simulink model "eTRU_prototype_2"  (R2021b)
settings: Solver=daessc  StartTime=0.0  StopTime=5000  MaxStep=1  RelTol=1e-2  AbsTol=1e-2
PostLoadFcn:
  | eTRU_prototype_2_init
InitFcn:
  | eTRU_prototype_2_start_sim
StartFcn:
  | tic
StopFcn:
  | toc
  | PlotSimResults
values from neighbouring files (symbols this model uses):
  AirFlow = [0 0 0 0 0 0 0 0 0 0;      2205 1950 1701 1679 1297 658 0 0 0 0;      2989 2767 2610 2594 2410 2343 2274 1771 0 0;      3704 3545 3432 3422 3307 3266 3216 2958 2888 2215]    [EC_FanData.m]
  ambient_temp = 20    [eTRU_prototype_2_start_sim.m]
  asm = block.DialogPrm(1).Data    [msfcn_StaticASM.m]
  box_start_temp = 20    [eTRU_prototype_2_start_sim.m]
  cargo_start_temp = box_start_temp    (= 20)    [eTRU_prototype_2_start_sim.m]
  Power = [5 5 5 5 5 5 5 5 5 5;      185 203 227 226 229 230 231 237 239 247;      420 442 458 461 496 509 522 528 530 538;      764 811 844 846 880 892 905 969 987 989]    [EC_FanData.m]
  Pressure = LimitValue(Pressure + LimitValue(Error/dvdP, -0.1, 0.1), obj.PressureMin/100000, obj.PressureMax/100000)    [CoolPropPyWrapper.m]    (also in EC_FanData.m = [0,127,217,225,316,349,383,559,607,865])
  Speed = [0,1840,2450,3060]    [EC_FanData.m]
libraries: fl_lib x109, nesl_utility x82, simulink_extras x13, SimscapeFluids_lib x4
(part 1 of 3)
settings Model: Creator=kks  LastModifiedBy=kaspe
settings SolverCC: MaxConsecutiveMinStep=1000  AlgebraicLoopSolver=TrustRegion
settings DataIOCC: SaveState=on
settings DebuggingCC: ReadBeforeWriteMsg=DisableAll  WriteAfterWriteMsg=DisableAll  WriteAfterReadMsg=DisableAll  MultiTaskDSMMsg=none  SFMachineParentedDataDiag=warning
settings ModelReferenceCC: UpdateModelReferenceTargets=IfOutOfDate
settings SFSimCC: SFSimEcho=off
settings SimscapeCC: SimscapeLogLimitData=off

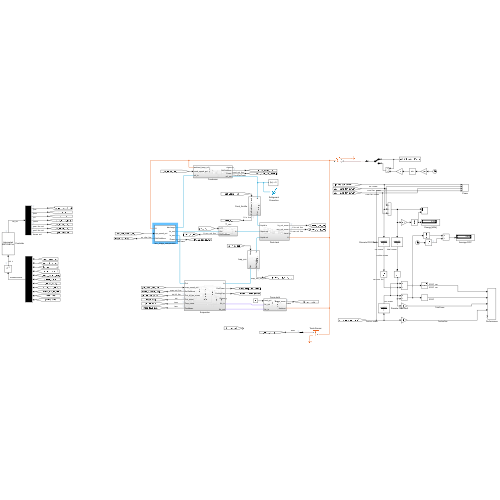
[thumbnail: Simulink's stored preview of the top-level diagram]
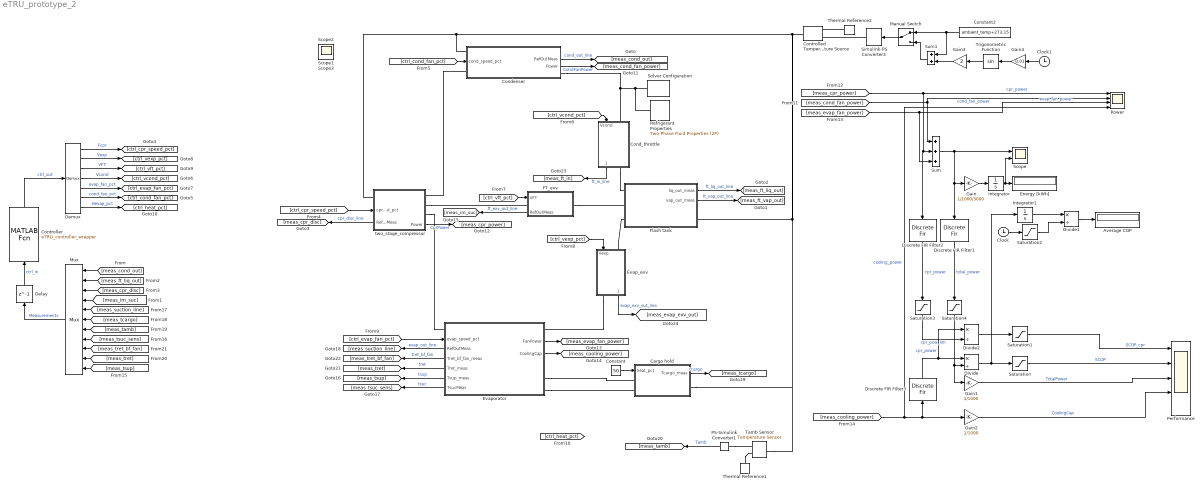
== system eTRU_prototype_2 ==
  Average COP : Display
  Cargo hold : Subsystem
  Clock : Clock
  Clock1 : Clock
  Cond_throttle : Subsystem
  Condenser : Subsystem
      settings: PortSchema="{\"entries\":[{\"content\":{\"sides\":[{\"content\":{\"connectorIds\":[\"LConn1\",\"In1\",\"LConn2\"]},\"type\":\"ConnectorPlacement.EquallySpacedRectSide\",\"uuid\":\"3d48dd4d-d64c-4c15-b87d-785ca519fd3e\"},{\"content\":{\"connectorIds\":[\"RConn1\",\"Out1\",\"Out2\",\"RConn2\"],\"side\":\"RIGHT\"},\"type\":\"ConnectorPlacement.EquallySpacedRectSide\",\"uuid\":\"adb43978-d4cf-4a53-b69c-b8e1726fc973\"},{\"content\":{\"connectorIds\":[],\"side\":\"TOP\"},\"type\":\"ConnectorPlacement.EquallySpacedRectSide\",\"uuid\":\"eda02cea-398b-4f5b-b755-168cdb387b03\"}]},\"type\":\"ConnectorPlacement.EquallySpacedConnector\",\"uuid\":\"bc915acd-4d9f-4179-86b8-14e03912b6e2\"}],\"packageUris\":[\"http://schema.mathworks.com/mf0/Connector/19700101\"],\"version\":\"1.0\"}"
  Constant : Constant  Value=50
  Constant2 : Constant  Value=ambient_temp+273.15
  Controlled Temperature Source : fl_lib/Thermal/Thermal Sources/Controlled Temperature Source
  Controller : MATLABFcn  StartFcn=eTRU_prototype_2_start_sim  MATLABFcn=eTRU_controller_wrapper
  Delay : Delay  DelayLength=1  InitialCondition=0  SampleTime=1
  Demux : Demux  Outputs=7
  Discrete FIR Filter1 : DiscreteFir  Coefficients=ones(1,300)/300
  Discrete FIR Filter2 : DiscreteFir  Coefficients=ones(1,300)/300
  Discrete FIR Filter3 : DiscreteFir  Coefficients=ones(1,300)/300
  Divide : Product  Inputs=*/
  Divide1 : Product  Inputs=*/
  Divide2 : Product  Inputs=*/
  Energy [kWh] : Display
  Evap_exv : Subsystem
      settings: PortSchema="{\"entries\":[{\"content\":{\"sides\":[{\"content\":{\"connectorIds\":[\"In1\",\"LConn1\"]},\"type\":\"ConnectorPlacement.EquallySpacedRectSide\",\"uuid\":\"a5f6ab4e-c003-4b63-bc8d-93a191bbc7b1\"},{\"content\":{\"connectorIds\":[\"RConn1\",\"Out1\"],\"side\":\"RIGHT\"},\"type\":\"ConnectorPlacement.EquallySpacedRectSide\",\"uuid\":\"60081e7c-9034-44ee-b85a-7fac1643604f\"},{\"content\":{\"connectorIds\":[],\"side\":\"TOP\"},\"type\":\"ConnectorPlacement.EquallySpacedRectSide\",\"uuid\":\"44f742ed-3697-4889-bc61-109290b38d73\"}]},\"type\":\"ConnectorPlacement.EquallySpacedConnector\",\"uuid\":\"b280b62a-8ac3-4a4b-85e3-fe929e92acc5\"}],\"packageUris\":[\"http://schema.mathworks.com/mf0/Connector/19700101\"],\"version\":\"1.0\"}"
  Evaporator : Subsystem
      settings: PortSchema="{\"entries\":[{\"content\":{\"sides\":[{\"content\":{\"connectorIds\":[\"LConn1\",\"In1\",\"Out3\",\"Out4\",\"Out5\",\"Out6\",\"Out7\"]},\"type\":\"ConnectorPlacement.EquallySpacedRectSide\",\"uuid\":\"033e4ee9-ae46-49ce-a29c-cb5691fe85b1\"},{\"content\":{\"connectorIds\":[\"RConn1\",\"Out1\",\"Out2\",\"RConn2\",\"RConn3\",\"RConn4\"],\"side\":\"RIGHT\"},\"type\":\"ConnectorPlacement.EquallySpacedRectSide\",\"uuid\":\"f5a957f7-d19d-4090-8dc6-9509ce363ce4\"},{\"content\":{\"connectorIds\":[],\"side\":\"TOP\"},\"type\":\"ConnectorPlacement.EquallySpacedRectSide\",\"uuid\":\"205ae6f2-ec5f-44bf-8412-6f03b41c638f\"},{\"content\":{\"connectorIds\":[],\"side\":\"BOTTOM\"},\"type\":\"ConnectorPlacement.EquallySpacedRectSide\",\"uuid\":\"b2e4c10a-8ecc-4b98-af22-93916696f813\"}]},\"type\":\"ConnectorPlacement.EquallySpacedConnector\",\"uuid\":\"b34f6f4b-92a6-4590-84b6-895e3d79e9bc\"}],\"packageUris\":[\"http://schema.mathworks.com/mf0/Connector/19700101\"],\"version\":\"1.0\"}"
  FT_exv : Subsystem
      settings: PortSchema="{\"entries\":[{\"content\":{\"sides\":[{\"content\":{\"connectorIds\":[\"LConn1\"]},\"type\":\"ConnectorPlacement.EquallySpacedRectSide\",\"uuid\":\"b279e9a8-1d21-4470-93a8-fbc83ce7b0b2\"},{\"content\":{\"connectorIds\":[\"In1\",\"RConn1\",\"Out1\"],\"side\":\"RIGHT\"},\"type\":\"ConnectorPlacement.EquallySpacedRectSide\",\"uuid\":\"0dfd93ae-010b-42e4-9e53-34ca9fdad0fd\"},{\"content\":{\"connectorIds\":[],\"side\":\"TOP\"},\"type\":\"ConnectorPlacement.EquallySpacedRectSide\",\"uuid\":\"f2d96627-f93b-40b5-bdbb-54ea25241c46\"}]},\"type\":\"ConnectorPlacement.EquallySpacedConnector\",\"uuid\":\"5e92ae64-a64b-485f-9000-97fefa6ea4c6\"}],\"packageUris\":[\"http://schema.mathworks.com/mf0/Connector/19700101\"],\"version\":\"1.0\"}"
  Flash tank : Subsystem
  Gain : Gain  Gain=1/1000/3600
  Gain1 : Gain  Gain=1/1000
  Gain2 : Gain  Gain=1/1000
  Gain3 : Gain  Gain=2
  Gain4 : Gain  Gain=0.01
  Integrator : Integrator
  Integrator1 : Integrator
  Manual Switch : ManualSwitch
  Mux : Mux  Inputs=11
  PS-Simulink Converter1 : nesl_utility/PS-Simulink Converter  PhysicalDomain=network_engine_domain  SubClassName=ps_output  LeftPortType=input  RightPortType=output  PseudoPeriodic=off  Frequencies=[]  Unit=inherit  AffineConversion=off
      settings: SourceProductBaseCode=PW,SS
  Performance : Scope  NumInputPorts=5
  Power : Scope  NumInputPorts=4
  Refrigerant Properties : fl_lib/Two-Phase Fluid/Utilities/Two-Phase Fluid Properties (2P)  u_min=RefrigerantPropertyTables.u_min kJ/kg  u_max=RefrigerantPropertyTables.u_max kJ/kg  p_TLU=RefrigerantPropertyTables.p MPa  p_crit=RefrigerantPropertyTables.p_crit MPa  critical_region=foundation.enum.critical_region.clip  p_crit_fraction=0.12  p_atm=0.101325 MPa  q_rev=0.01 Pa  unorm_liq=RefrigerantPropertyTables.liquid.unorm  v_liq=RefrigerantPropertyTables.liquid.v m^3/kg  s_liq=RefrigerantPropertyTables.liquid.s kJ/(K*kg)  T_liq=RefrigerantPropertyTables.liquid.T K  nu_liq=RefrigerantPropertyTables.liquid.nu mm^2/s  k_liq=RefrigerantPropertyTables.liquid.k W/(m*K)  Pr_liq=RefrigerantPropertyTables.liquid.Pr  u_sat_liq=RefrigerantPropertyTables.liquid.u_sat kJ/kg  unorm_vap=RefrigerantPropertyTables.vapor.unorm  v_vap=RefrigerantPropertyTables.vapor.v m^3/kg  s_vap=RefrigerantPropertyTables.vapor.s kJ/(K*kg)  T_vap=RefrigerantPropertyTables.vapor.T K  nu_vap=RefrigerantPropertyTables.vapor.nu mm^2/s  k_vap=RefrigerantPropertyTables.vapor.k W/(m*K)  Pr_vap=RefrigerantPropertyTables.vapor.Pr  u_sat_vap=RefrigerantPropertyTables.vapor.u_sat kJ/kg
      settings: SourceProductBaseCode=SS  InternalSimscapePortConfiguration="{\"Bottom\":[],\"Left\":[],\"Right\":[{\"id\":\"A\",\"label\":\"\",\"type\":\"foundation.two_phase_fluid.two_phase_fluid\"}],\"Top\":[]}"
  Saturation : Saturate  UpperLimit=10  LowerLimit=0
  Saturation1 : Saturate  UpperLimit=10  LowerLimit=0
  Saturation2 : Saturate  UpperLimit=20000000  LowerLimit=0.0001
  Saturation3 : Saturate  UpperLimit=20000  LowerLimit=0.0001
  Saturation4 : Saturate  UpperLimit=20000  LowerLimit=0.0001
  Scope : Scope  NumInputPorts=2
  Simulink-PS Converter3 : nesl_utility/Simulink-PS Converter  PhysicalDomain=network_engine_domain  SubClassName=ps_input  LeftPortType=input  RightPortType=output  PseudoPeriodic=off  Frequencies=[]  NoiseDistribution=none  NoiseParameters=[]  Unit=K  AffineConversion=off  FilteringAndDerivatives=zero  SimscapeFilterOrder=1  InputFilterTimeConstant=0.001  UdotUserProvided=1
      settings: SourceProductBaseCode=PW,SS
  Solver Configuration : nesl_utility/Solver Configuration  PhysicalDomain=network_engine_domain  SubClassName=solver  LeftPortType=input  RightPortType=generic  Tones=[]  Harmonics=[]  SimulateNoise=off  Profile=off  UseLocalSampling=off  EnableSwitchedLinearOptims=on  FrequencyDomain=off  UseCCode=off  RelTol=0.001  AbsTol=1e-06  MinStep=1e-09  ToWorkspace=off  RevertToSquareIcSolve=off  NumHomotopyIterations=100  PhasorMode=off  PhasorModeNumHarmonics=1  DoDC=off  ResidualTolerance=1e-3  UseLocalSolver=off  LocalSolverChoice=NE_BACKWARD_EULER_ADVANCER  LocalSolverSampleTime=.01  DoFixedCost=off  MaxNonlinIter=3  MaxModeIter=2  ComputeImpulses=off  ImpulseIterations=2  LinearAlgebra=auto  EquationFormulation=NE_TIME_EF  DelaysMemoryBudget=1024  AutomaticFiltering=on  FilteringTimeConstant=0.001  PartitionStorageMethod=AS_NEEDED  PartitionMemoryBudget=1024  PartitionMethod=FAST
      settings: SourceProductBaseCode=PW,SS
  Sum : Sum  Inputs=+++
  Sum1 : Sum
  Tamb Sensor : fl_lib/Thermal/Thermal Sensors/Temperature Sensor
  Thermal Reference1 : fl_lib/Thermal/Thermal Elements/Thermal Reference
  Thermal Reference2 : fl_lib/Thermal/Thermal Elements/Thermal Reference
  Trigonometric Function : Trigonometry
  two_stage_compressor : Subsystem
      settings: PortSchema="{\"entries\":[{\"content\":{\"sides\":[{\"content\":{\"connectorIds\":[\"LConn1\",\"In1\",\"Out2\"]},\"type\":\"ConnectorPlacement.EquallySpacedRectSide\",\"uuid\":\"3d48dd4d-d64c-4c15-b87d-785ca519fd3e\"},{\"content\":{\"connectorIds\":[\"RConn1\",\"RConn2\",\"RConn3\",\"Out1\"],\"side\":\"RIGHT\"},\"type\":\"ConnectorPlacement.EquallySpacedRectSide\",\"uuid\":\"adb43978-d4cf-4a53-b69c-b8e1726fc973\"},{\"content\":{\"connectorIds\":[],\"side\":\"TOP\"},\"type\":\"ConnectorPlacement.EquallySpacedRectSide\",\"uuid\":\"eda02cea-398b-4f5b-b755-168cdb387b03\"},{\"content\":{\"connectorIds\":[],\"side\":\"BOTTOM\"},\"type\":\"ConnectorPlacement.EquallySpacedRectSide\",\"uuid\":\"387ca0a5-5948-431b-aa88-e67186ab9723\"}]},\"type\":\"ConnectorPlacement.EquallySpacedConnector\",\"uuid\":\"bc915acd-4d9f-4179-86b8-14e03912b6e2\"}],\"packageUris\":[\"http://schema.mathworks.com/mf0/Connector/19700101\"],\"version\":\"1.0\"}"
  Scope1 : Scope
  Scope2 : Scope
  Scope3 : Scope
  wires:
  Mux/1 -> Delay/1  "Measurements"
  Controller/1 -> Demux/1  "ctrl_out"
  Delay/1 -> Controller/1  "ctrl_in"
  [meas_cond_out] -> Mux/1
  [meas_im_suc] -> Mux/4
  [meas_ft_liq_out] -> Mux/2
  [meas_cpr_disc] -> Mux/3
  Integrator/1 -> Scope/2, Energy [kWh]/1
  Gain/1 -> Integrator/1
  Divide/1 -> Integrator1/1, Saturation/1
  Gain1/1 -> Performance/3  "TotalPower"
  Gain2/1 -> Performance/4  "CoolingCap"
  Sum/1 -> Discrete FIR Filter1/1, Gain/1, Scope/1
  Flash tank/1(liq_out_meas) -> [meas_ft_liq_out]  "ft_liq_out_line"
  Flash tank/2(vap_out_meas) -> [meas_ft_vap_out]  "ft_vap_out_line"
  Condenser/1(RefOutMeas) -> [meas_cond_out]  "cond_out_line"
  two_stage_compressor/2(RefOutMeas) -> [meas_cpr_disc]  "cpr_disc_line"
  Demux/1 -> [ctrl_cpr_speed_pct]  "Fcpr"
  [ctrl_cpr_speed_pct] -> two_stage_compressor/1(cpr_speed_pct)
  [ctrl_cond_fan_pct] -> Condenser/1(cond_speed_pct)
  Demux/6 -> [ctrl_cond_fan_pct]  "cond_fan_pct"
  [ctrl_vcond_pct] -> Cond_throttle/1(Vcond)
  Demux/4 -> [ctrl_vcond_pct]  "Vcond"
  [ctrl_evap_fan_pct] -> Evaporator/1(evap_speed_pct)
  Demux/5 -> [ctrl_evap_fan_pct]  "evap_fan_pct"
  [ctrl_vexp_pct] -> Evap_exv/1(Vexp)
  [ctrl_vft_pct] -> FT_exv/1(VFT)
  Demux/2 -> [ctrl_vexp_pct]  "Vexp"
  Demux/3 -> [ctrl_vft_pct]  "VFT"
  Demux/7 -> [ctrl_heat_pct]  "Hevap_pct"
  Condenser/2(Power) -> [meas_cond_fan_power]  "CondFanPower"
  [meas_cond_fan_power] -> Sum/1, Power/2  "cond_fan_power"
  two_stage_compressor/1(Power) -> [meas_cpr_power]  "CprPower"
  [meas_cpr_power] -> Discrete FIR Filter2/1, Sum/2, Power/1  "cpr_power"
  [meas_evap_fan_power] -> Sum/3, Power/3  "evap_fan_power"
  Evaporator/1(FanPower) -> [meas_evap_fan_power]
  Evaporator/2(CoolingCap) -> [meas_cooling_power]
  [meas_cooling_power] -> Discrete FIR Filter3/1, Gain2/1, Power/4  "cooling_power"
  FT_exv/1(RefOutMeas) -> [meas_im_suc]  "ft_exv_out_line"
  Evaporator/3(RefOutMeas) -> [meas_suction_line]  "evap_out_line"
  [meas_suction_line] -> Mux/5
  Evaporator/7(TsucMeas) -> [meas_tsuc_sens]  "tsuc"
  [meas_tsuc_sens] -> Mux/8
  PS-Simulink Converter1/1 -> [meas_tamb]  "Tamb"
  [meas_tamb] -> Mux/7
  [meas_tcargo] -> Mux/6
  Cargo hold/1(Tcargo_meas) -> [meas_tcargo]  "tcargo"
  Evaporator/4(Tret_bf_fan_meas) -> [meas_tret_bf_fan]  "tret_bf_fan"
  [meas_tret_bf_fan] -> Mux/9
  Evaporator/5(Tret_meas) -> [meas_tret]  "tret"
  [meas_tret] -> Mux/10
  Evaporator/6(Tsup_meas) -> [meas_tsup]  "tsup"
  [meas_tsup] -> Mux/11
  Cond_throttle/1(RefOutMeas) -> [meas_ft_in]  "ft_in_line"
  Evap_exv/1(RefOutMeas) -> [meas_evap_exv_out]  "evap_exv_out_line"
  Clock/1 -> Saturation2/1
  Integrator1/1 -> Divide1/1
  Divide1/1 -> Average COP/1
  Saturation1/1 -> Performance/1  "SCOP_cpr"
  Clock1/1 -> Gain4/1
  Manual Switch/1 -> Simulink-PS Converter3/1
  Constant2/1 -> Manual Switch/1, Sum1/1
  Trigonometric Function/1 -> Gain3/1
  Sum1/1 -> Manual Switch/2
  Gain3/1 -> Sum1/2
  Gain4/1 -> Trigonometric Function/1
  Saturation3/1 -> Divide2/2  "cpr_pow_lim"
  Saturation4/1 -> Divide/2, Gain1/1
  Discrete FIR Filter2/1 -> Saturation3/1  "cpr_power"
  Discrete FIR Filter1/1 -> Saturation4/1  "total_power"
  Divide2/1 -> Saturation1/1
  Saturation/1 -> Performance/2  "SCOP"
  Saturation2/1 -> Divide1/2
  Discrete FIR Filter3/1 -> Divide/1, Divide2/1  "cpr_power"
  Constant/1 -> Cargo hold/1(heat_pct)
  connections:
  Solver Configuration/RConn1 -- Refrigerant Properties/RConn1 -- Condenser/RConn2 -- Cond_throttle/LConn1
  two_stage_compressor/LConn1 -- Flash tank/RConn2 -- Cargo hold/RConn1 -- Tamb Sensor/LConn1 -- Controlled Temperature Source/LConn1 -- Condenser/LConn1
  two_stage_compressor/RConn2 -- FT_exv/RConn1
  two_stage_compressor/RConn3 -- Evaporator/LConn1
  Thermal Reference1/LConn1 -- Tamb Sensor/RConn1
  PS-Simulink Converter1/LConn1 -- Tamb Sensor/RConn2
  Evap_exv/RConn1 -- Evaporator/RConn1
  Evaporator/RConn3 -- Cargo hold/LConn1
  Evaporator/RConn4 -- Cargo hold/LConn2
  FT_exv/LConn1 -- Flash tank/LConn2
  Evap_exv/LConn1 -- Flash tank/LConn3
  Cond_throttle/RConn1 -- Flash tank/LConn1
  Condenser/LConn2 -- two_stage_compressor/RConn1
  Simulink-PS Converter3/RConn1 -- Controlled Temperature Source/RConn1
  Thermal Reference2/LConn1 -- Controlled Temperature Source/RConn2

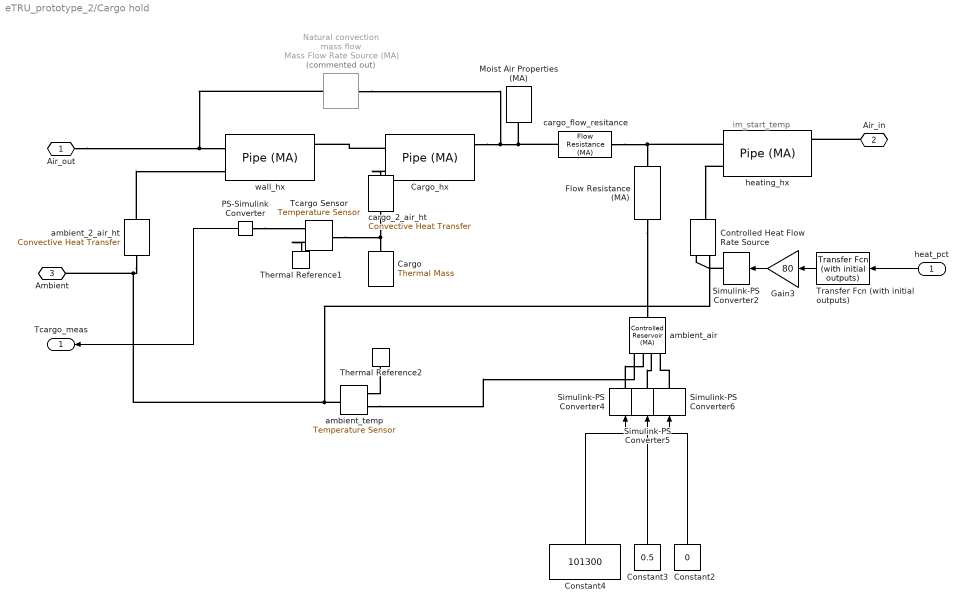
== system eTRU_prototype_2/Cargo hold ==
  note: im_start_temp
  heat_pct : Inport
  Cargo : fl_lib/Thermal/Thermal Elements/Thermal Mass  mass=cargo_mass kg  sp_heat=447 J/kg/K  T_specify=on  T_priority=Low  T=cargo_start_temp degC  T_nominal_specify=off  T_nominal_unit=K  T_nominal_value=1  Q_specify=off  Q_priority=None  Q=0 W  Q_nominal_specify=off  Q_nominal_unit=W  Q_nominal_value=1
  Cargo_hx : fl_lib/Moist Air/Elements/Pipe (MA)  length=12 m  area=2.5*2.5 m^2  Dh=0.1 m  length_add=0.1 m  roughness=15e-6 m  Re_lam=2000  Re_tur=4000  shape_factor=64  Nu_lam=3.66  RH_ws=1  time_constant=1e-3 s  moisture_trace_gas_source=foundation.enum.moisture_trace_gas_source.none  moisture_source_spec=foundation.enum.moisture_source_spec.vapor  moisture_mass_flow=0 kg/s  moisture_temperature_spec=foundation.enum.temperature_spec.atmospheric  moisture_temperature=293.15 K  trace_gas_mass_flow=0 kg/s  trace_gas_temperature_spec=foundation.enum.temperature_spec.atmospheric  trace_gas_temperature=293.15 K  p_I_specify=off  p_I_priority=High  p_I=0.101325 MPa  p_I_nominal_specify=off  p_I_nominal_unit=MPa  p_I_nominal_value=1  T_I_specify=on  T_I_priority=High  T_I=box_start_temp degC  T_I_nominal_specify=off  T_I_nominal_unit=K  T_I_nominal_value=1  RH_I_specify=on  RH_I_priority=High  RH_I=0.5  RH_I_nominal_specify=off  RH_I_nominal_unit=1  RH_I_nominal_value=1  x_w_I_specify=off  x_w_I_priority=None  x_w_I=0  x_w_I_nominal_specify=off  x_w_I_nominal_unit=1  x_w_I_nominal_value=1  y_w_I_specify=off  y_w_I_priority=None  y_w_I=0  y_w_I_nominal_specify=off  y_w_I_nominal_unit=1  y_w_I_nominal_value=1  HR_I_specify=off  HR_I_priority=None  HR_I=0  HR_I_nominal_specify=off  HR_I_nominal_unit=1  HR_I_nominal_value=1  x_g_I_specify=off  x_g_I_priority=High  x_g_I=0  x_g_I_nominal_specify=off  x_g_I_nominal_unit=1  x_g_I_nominal_value=1  y_g_I_specify=off  y_g_I_priority=None  y_g_I=0  y_g_I_nominal_specify=off  y_g_I_nominal_unit=1  y_g_I_nominal_value=1
      settings: SourceProductBaseCode=SS
  Constant2 : Constant  Value=0
  Constant3 : Constant  Value=0.5
  Constant4 : Constant  Value=101300
  Controlled Heat Flow Rate Source : fl_lib/Thermal/Thermal Sources/Controlled Heat Flow Rate Source
  Flow Resistance (MA) : fl_lib/Moist Air/Elements/Flow Resistance (MA)  delta_p_nominal=0.1 MPa  mdot_nominal=0.1 kg/s  rho_nominal=0 kg/m^3  area=0.01 m^2  laminar_fraction=1e-3
      settings: SourceProductBaseCode=SS
  Gain3 : Gain  Gain=80
  Moist Air Properties (MA) : fl_lib/Moist Air/Utilities/Moist Air Properties (MA)  R_a=287.047 J/kg/K  T_TLU=[-56.55, -50 : 10 : -10, -5 : 1 : 5, 10 : 10 : 350]' degC  h_a_TLU=[342.416126230579; 349.005511058471; 359.063577249119; 369.119948684177; 379.175469465129; 389.230944678417; 394.258910928084; 395.264534937366; 396.27017101329; 397.275819932805; 398.281482472874; 399.287159410541; 400.292851523015; 401.298559587728; 402.304284382408; 403.310026685143; 404.315787274435; 409.34489180313; 419.404921755863; 429.468036401264; 439.535033154839; 449.606720928652; 459.683919949603; 469.767460521911; 479.858181001348; 489.956925196484; 500.064539372946; 510.181869006204; 520.309755403634; 530.449032296018; 540.60052248087; 550.765034584465; 560.943359995745; 571.136270013102; 581.344513234296; 591.568813210327; 601.809866375885; 612.068340261954; 622.344871990218; 632.640067043998; 642.95449830646; 653.288705353699; 663.643193987949; 674.018435994423; 684.414869104228; 694.832897145098; 705.272890361557; 715.735185886199; 726.220088344236; 736.727870574087; 747.258774447567; 757.813011774199] kJ/kg  mu_a_TLU=[14.2568883320012; 14.6140127728333; 15.1517277055779; 15.6806860159119; 16.2012351072083; 16.7137043125028; 16.9670071730589; 17.017438062815; 17.0677930842452; 17.1180725309876; 17.1682766951315; 17.2184058672268; 17.2684603362935; 17.3184403898301; 17.3683463138234; 17.4181783927569; 17.4679369096204; 17.7156358640698; 18.2056751785154; 18.68879035749; 19.1652344664982; 19.6352478927873; 20.099059103658; 20.5568853601578; 21.0089333871663; 21.4554000014051; 21.8964726992323; 22.3323302062775; 22.7631429910631; 23.1890737447833; 23.6102778293792; 24.0269036959922; 24.4390932757886; 24.8469823450548; 25.2507008663546; 25.6503733074314; 26.0461189394339; 26.4380521159325; 26.8262825340948; 27.2109154792923; 27.5920520543128; 27.969789394274; 28.3442208682439; 28.7154362685068; 29.0835219883356; 29.4485611890712; 29.8106339572472; 30.1698174524429; 30.5261860464955; 30.8798114546565; 31.2307628592324; 31.5791070262086] s*uPa  k_a_TLU=[19.8808489374933; 20.4162454629695; 21.2248743590758; 22.0232452890903; 22.8117314495857; 23.5906913619588; 23.9767075412237; 24.053639990175; 24.1304826682191; 24.2072359051629; 24.2839000294007; 24.3604753679152; 24.4369622462801; 24.5133609886625; 24.5896719178249; 24.6658953551279; 24.7420316205333; 25.1214164701832; 25.8738283029331; 26.6180150229276; 27.3542674377332; 28.0828634735341; 28.8040686837224; 29.5181367785657; 30.2253101618423; 30.9258204644224; 31.6198890677835; 32.3077276126633; 32.9895384896798; 33.6655153099498; 34.33584335461; 35.0007000027879; 35.6602551380254; 36.3146715334901; 36.9641052165342; 37.6087058133173; 38.248616874307; 38.8839761815308; 39.5149160384798; 40.1415635435708; 40.7640408480637; 41.3824653993118; 41.9969501701893; 42.6076038755117; 43.2145311762238; 43.8178328720941; 44.4176060836121; 45.013944423749; 45.6069381602018; 46.1966743687041; 46.783237077953; 47.3667074066625] mW/m/K  p_min=1 kPa  p_max=inf MPa  T_min=-56.55 degC  T_max=350 degC  p_atm=0.101325 MPa  T_atm=20 degC  R_w=461.523 J/kg/K  p_ws_TLU=[1.71168953425982e-06; 3.93770601979424e-06; 1.28411717710344e-05; 3.80051394873809e-05; .00010323902900209; .000259873810798063; .000401741022116384; .000437454836117844; .000476040820618202; .000517704666185737; .000562664883741207; .000611212677444345; .000657088049117899; .000705987905898279; .000758082381149132; .000813549384183233; .000872574861129522; .00122818386934022; .0023392147667769; .00424668834054807; .00738442748706953; .0123512704340234; .0199458019246787; .0312006356960619; .0474147199263783; .0701823607447713; .10141797792131; .143375967241115; .198665399739302; .270259606559999; .361500961984849; .476101381081492; .618139196722055; .792053183687694; 1.0026345688121; 1.25501792086105; 1.55467186826983; 1.90739066433297; 2.31928772772542; 2.79679245576864; 3.34665187151016; 3.97593907083533; 4.69207105435535; 5.5028394740883; 6.41645928168037; 7.4416425436169; 8.58770832955728; 9.86474556030261; 11.2838558865497; 12.8575218898034; 14.6001810568052; 16.5291642526045] MPa  h_w_vap_TLU=[2836.88241275372; 2837.81392500514; 2838.63937175807; 2838.7309929628; 2838.06905313927; 2836.62597341095; 2835.60023952573; 2835.37006381376; 2835.13143158077; 2834.88429145066; 2834.62859062897; 2500.93420564316; 2498.55329907119; 2496.17495082036; 2493.79885912205; 2491.42474723191; 2489.05236104642; 2477.20875029194; 2453.54955988604; 2429.83856603313; 2406.00136954922; 2381.97406342174; 2357.69101156389; 2333.08088387814; 2308.06565480412; 2282.56034405021; 2256.47287422313; 2229.70428017508; 2202.14968030993; 2173.69998896199; 2144.24368406447; 2113.66758247452; 2081.85585110571; 2048.68725710494; 2014.03141249899; 1977.7449923284; 1939.66849592886; 1899.62342931686; 1857.40930169838; 1812.79975416601; 1765.53721731251; 1715.32525772152; 1661.81700477787; 1604.59703745016; 1543.1534616334; 1476.83692476464; 1404.80240352424; 1325.92091736114; 1238.61667822208; 1140.5102987018; 1027.62017777647; 892.733785613825] kJ/kg  h_w_TLU=[2396.55944251649; 2408.68643343608; 2427.1988031141; 2445.702165897; 2464.18429108356; 2482.62529466839; 2491.82135326629; 2493.6580151792; 2495.49372578218; 2497.32843835745; 2499.16210446923; 2500.99462758899; 2502.83092214066; 2504.6665223621; 2506.50140563013; 2508.335548891; 2510.16892865793; 2519.32352241995; 2537.56068088674; 2555.67742615292; 2573.6403223998; 2591.4109179101; 2608.9455037701; 2626.19492016262; 2643.10444358428; 2659.61377634497; 2675.58278696023; 2696.1846256545; 2716.49989553741; 2736.6235210957; 2756.61216047011; 2776.50561773853; 2796.33378922508; 2816.11979583049; 2835.88181423877; 2855.63430574511; 2875.38889327595; 2895.15500577172; 2914.94035964689; 2934.75132290228; 2954.59319330244; 2974.47041285505; 2994.38673458964; 3014.34535328009; 3034.34900867103; 3054.40006755764; 3074.50058946898; 3094.65237953784; 3114.85703128106; 3135.11596137801; 3155.43043805905; 3175.80160435813] kJ/kg  mu_w_TLU=[6.81365662228272; 7.04953750742707; 7.40970098298307; 7.76991278093907; 8.13017290129507; 8.49048134405107; 8.67065368632907; 8.70668960445667; 8.74272600580827; 8.77876289038387; 8.81480025818347; 8.85083810920707; 8.88687644345467; 8.92291526092627; 8.95895456162187; 8.99499434554147; 9.03103461268507; 9.21124319676307; 9.57169660671907; 9.93219833907507; 10.2927483938311; 10.6533467709871; 11.0139934705431; 11.3746884924991; 11.7354318368551; 12.0962235036111; 12.4570634927671; 12.8179518043231; 13.1788884382791; 13.5398733946351; 13.9009066733911; 14.2619882745471; 14.6231181981031; 14.9842964440591; 15.3455230124151; 15.7067979031711; 16.0681211163271; 16.4294926518831; 16.7909125098391; 17.1523806901951; 17.5138971929511; 17.8754620181071; 18.2370751656631; 18.5987366356191; 18.9604464279751; 19.3222045427311; 19.6840109798871; 20.0458657394431; 20.4077688213991; 20.7697202257551; 21.1317199525111; 21.4937680016671] s*uPa  k_w_TLU=[11.46288215976; 11.941997488935; 12.676358586935; 13.414208884935; 14.155548382935; 14.900377080935; 15.274099879935; 15.348949115735; 15.423833243535; 15.498752263335; 15.573706175135; 15.648694978935; 15.723718674735; 15.798777262535; 15.873870742335; 15.948999114135; 16.024162377935; 16.400502076935; 17.155798374935; 17.914583872935; 18.676858570935; 19.442622468935; 20.211875566935; 20.984617864935; 21.760849362935; 22.540570060935; 23.323779958935; 24.110479056935; 24.900667354935; 25.694344852935; 26.491511550935; 27.292167448935; 28.096312546935; 28.903946844935; 29.715070342935; 30.529683040935; 31.347784938935; 32.169376036935; 32.994456334935; 33.823025832935; 34.655084530935; 35.490632428935; 36.329669526935; 37.172195824935; 38.018211322935; 38.867716020935; 39.720709918935; 40.577193016935; 41.437165314935; 42.300626812935; 43.167577510935; 44.038017408935] mW/m/K  D_w=25 mm^2/s  trace_gas_model=foundation.enum.trace_gas_model.none  R_g=188.923 J/kg/K  h_g_TLU=[439.555216260064; 444.670268200251; 452.538618847003; 460.487124258496; 468.522588768941; 476.649415958793; 480.74798538725; 481.57054318762; 482.394052398751; 483.218514288831; 484.043930029015; 484.870300696555; 485.697627277859; 486.525910671489; 487.355151691079; 488.185351068185; 489.016509455051; 493.186704139431; 501.599194953048; 510.107689961685; 518.711611080182; 527.410026793075; 536.201764778798; 545.085474203452; 554.059675505208; 563.122805485367; 572.27325096919; 581.509373027928; 590.829525105886; 600.232066705818; 609.715373581392; 619.277845178105; 628.917909922924; 638.634028838794; 648.424697859328; 658.288449140109; 668.223851601449; 678.229510889093; 688.304068901113; 698.44620299875; 708.654624994591; 718.928079991818; 729.265345132425; 739.665228299475; 750.126566808087; 760.648226111439; 771.229098541268; 781.868102096908; 792.564179292476; 803.316296068366; 814.123440770426; 824.984623198037] kJ/kg  mu_g_TLU=[10.8921054191698; 11.2215357085649; 11.7233300740382; 12.2234238147811; 12.7215124453467; 13.2173328890673; 13.4643203184773; 13.5136406274989; 13.562934752385; 13.6122025024997; 13.6614436900741; 13.7106581301692; 13.7598456406398; 13.8090060420983; 13.8581391578796; 13.9072448140062; 13.9563228391538; 14.2012926853717; 14.6890687376044; 15.1738428124161; 15.6554929043332; 16.1339159800463; 16.6090257998657; 17.0807510097148; 17.5490334645512; 18.0138267508952; 18.4750948814453; 18.9328111390399; 19.3869570507278; 19.8375214755778; 20.2844997922255; 20.7278931741254; 21.1677079421287; 21.6039549853963; 22.036649242835; 22.4658092382469; 22.8914566632375; 23.3136160026627; 23.7323141980278; 24.1475803447965; 24.5594454200432; 24.9679420372927; 25.3731042257492; 25.774967231431; 26.1735673380029; 26.5689417053362; 26.9611282240413; 27.350165384404; 27.73609215832; 28.118947892972; 28.4987722151178; 28.8756049449796] s*uPa  k_g_TLU=[10.489430678843; 10.9507672150864; 11.666197960308; 12.392559739764; 13.1299519771612; 13.8778409888416; 14.2554325416312; 14.3312274189707; 14.4071122346908; 14.4830860227061; 14.5591478179508; 14.6352966574703; 14.7115315815553; 14.787851634907; 14.8642558678259; 14.9407433374142; 15.0173131087819; 15.401364480906; 16.1751373988038; 16.9558134611595; 17.7432208682398; 18.5366976599676; 19.3360988502003; 20.1412225692689; 20.9517507672929; 21.7672310558863; 22.5871115634685; 23.4107980865695; 24.2377021890869; 25.0672663781241; 25.8989689893876; 26.732318357514; 27.5668446164644; 28.4020933015927; 29.2376215872816; 30.0729965057542; 30.9077942826816; 31.7416001931033; 32.5740086297993; 33.4046232539953; 34.2330571812868; 35.0589331874899; 35.8818839295189; 36.701552179391; 37.5175910702657; 38.3296643536716; 39.1374466671854; 39.9406238119064; 40.7388930391313; 41.5319633456945; 42.3195557774861; 43.1014037407076] mW/m/K  D_g=16 mm^2/s
      settings: SourceProductBaseCode=SS
  Natural convection mass flow : fl_lib/Moist Air/Sources/Mass Flow Rate Source (MA)  Commented=on  power_spec=foundation.enum.power_spec.none  mass_flow=0.1 kg/s  area_A=1 m^2  area_B=1 m^2
      settings: SourceProductBaseCode=SS  InternalSimscapePortConfiguration="{\"Bottom\":[],\"Left\":[{\"id\":\"A\",\"label\":\"A\",\"type\":\"foundation.moist_air.moist_air\"}],\"Right\":[{\"id\":\"B\",\"label\":\"B\",\"type\":\"foundation.moist_air.moist_air\"}],\"Top\":[]}"
  PS-Simulink Converter : nesl_utility/PS-Simulink Converter  PhysicalDomain=network_engine_domain  SubClassName=ps_output  LeftPortType=input  RightPortType=output  PseudoPeriodic=off  Frequencies=[]  Unit=inherit  AffineConversion=off
      settings: SourceProductBaseCode=PW,SS
  Simulink-PS Converter2 : nesl_utility/Simulink-PS Converter  PhysicalDomain=network_engine_domain  SubClassName=ps_input  LeftPortType=input  RightPortType=output  PseudoPeriodic=off  Frequencies=[]  NoiseDistribution=none  NoiseParameters=[]  Unit=W  AffineConversion=off  FilteringAndDerivatives=zero  SimscapeFilterOrder=1  InputFilterTimeConstant=0.001  UdotUserProvided=1
      settings: SourceProductBaseCode=PW,SS
  Simulink-PS Converter4 : nesl_utility/Simulink-PS Converter  PhysicalDomain=network_engine_domain  SubClassName=ps_input  LeftPortType=input  RightPortType=output  PseudoPeriodic=off  Frequencies=[]  NoiseDistribution=none  NoiseParameters=[]  Unit=Pa  AffineConversion=off  FilteringAndDerivatives=zero  SimscapeFilterOrder=1  InputFilterTimeConstant=0.001  UdotUserProvided=1
      settings: SourceProductBaseCode=PW,SS
  Simulink-PS Converter5 : nesl_utility/Simulink-PS Converter  PhysicalDomain=network_engine_domain  SubClassName=ps_input  LeftPortType=input  RightPortType=output  PseudoPeriodic=off  Frequencies=[]  NoiseDistribution=none  NoiseParameters=[]  Unit=Wb  AffineConversion=off  FilteringAndDerivatives=zero  SimscapeFilterOrder=1  InputFilterTimeConstant=0.001  UdotUserProvided=1
      settings: SourceProductBaseCode=PW,SS
  Simulink-PS Converter6 : nesl_utility/Simulink-PS Converter  PhysicalDomain=network_engine_domain  SubClassName=ps_input  LeftPortType=input  RightPortType=output  PseudoPeriodic=off  Frequencies=[]  NoiseDistribution=none  NoiseParameters=[]  Unit=kg/s  AffineConversion=off  FilteringAndDerivatives=zero  SimscapeFilterOrder=1  InputFilterTimeConstant=0.001  UdotUserProvided=1
      settings: SourceProductBaseCode=PW,SS
  Tcargo Sensor : fl_lib/Thermal/Thermal Sensors/Temperature Sensor
  Thermal Reference1 : fl_lib/Thermal/Thermal Elements/Thermal Reference
  Thermal Reference2 : fl_lib/Thermal/Thermal Elements/Thermal Reference
  Transfer Fcn (with initial outputs) : simulink_extras/Additional Linear/Transfer Fcn (with initial outputs)  N=[1]  D="[1  1]"  Y0=0  U0=0
  ambient_2_air_ht : fl_lib/Thermal/Thermal Elements/Convective Heat Transfer  area=12*2.5*2.5 m^2  heat_tr_coeff=0.6000 W/(m^2 * K)  T_specify=off  T_priority=None  T=0 K  T_nominal_specify=off  T_nominal_unit=K  T_nominal_value=1  Q_specify=off  Q_priority=None  Q=0 W  Q_nominal_specify=off  Q_nominal_unit=W  Q_nominal_value=1
  ambient_air : fl_lib/Moist Air/Elements/Controlled Reservoir (MA)  moisture_spec=foundation.enum.moisture_spec.relative_humidity  trace_gas_spec=foundation.enum.trace_gas_spec.mass_fraction  RH_ws=1  area_A=0.01 m^2  input_error_spec=foundation.enum.input_range_error.warn
      settings: SourceProductBaseCode=SS  InternalSimscapePortConfiguration="{\"Bottom\":[],\"Left\":[{\"id\":\"A\",\"label\":\"A\",\"type\":\"foundation.moist_air.moist_air\"}],\"Right\":[{\"id\":\"T\",\"label\":\"T\",\"type\":\"input\"},{\"id\":\"P\",\"label\":\"P\",\"type\":\"input\"},{\"id\":\"W\",\"label\":\"W\",\"type\":\"input\"},{\"id\":\"G\",\"label\":\"G\",\"type\":\"input\"}],\"Top\":[]}"
  ambient_temp : fl_lib/Thermal/Thermal Sensors/Temperature Sensor
  cargo_2_air_ht : fl_lib/Thermal/Thermal Elements/Convective Heat Transfer  area=100 m^2  heat_tr_coeff=20 W/(m^2 * K)  T_specify=off  T_priority=None  T=0 K  T_nominal_specify=off  T_nominal_unit=K  T_nominal_value=1  Q_specify=off  Q_priority=None  Q=0 W  Q_nominal_specify=off  Q_nominal_unit=W  Q_nominal_value=1
  cargo_flow_resitance : fl_lib/Moist Air/Elements/Flow Resistance (MA)  delta_p_nominal=400 Pa  mdot_nominal=1.7 kg/s  rho_nominal=0 kg/m^3  area=1 m^2  laminar_fraction=1e-3
      settings: SourceProductBaseCode=SS
  heating_hx : fl_lib/Moist Air/Elements/Pipe (MA)  length=12 m  area=2.5*2.5 m^2  Dh=2.5 m  length_add=0.1 m  roughness=15e-6 m  Re_lam=2000  Re_tur=4000  shape_factor=64  Nu_lam=3.66  RH_ws=1  time_constant=1e-3 s  moisture_trace_gas_source=foundation.enum.moisture_trace_gas_source.none  moisture_source_spec=foundation.enum.moisture_source_spec.vapor  moisture_mass_flow=0 kg/s  moisture_temperature_spec=foundation.enum.temperature_spec.atmospheric  moisture_temperature=293.15 K  trace_gas_mass_flow=0 kg/s  trace_gas_temperature_spec=foundation.enum.temperature_spec.atmospheric  trace_gas_temperature=293.15 K  p_I_specify=off  p_I_priority=High  p_I=0.101325 MPa  p_I_nominal_specify=off  p_I_nominal_unit=MPa  p_I_nominal_value=1  T_I_specify=on  T_I_priority=High  T_I=box_start_temp degC  T_I_nominal_specify=off  T_I_nominal_unit=K  T_I_nominal_value=1  RH_I_specify=on  RH_I_priority=High  RH_I=0.5  RH_I_nominal_specify=off  RH_I_nominal_unit=1  RH_I_nominal_value=1  x_w_I_specify=off  x_w_I_priority=None  x_w_I=0  x_w_I_nominal_specify=off  x_w_I_nominal_unit=1  x_w_I_nominal_value=1  y_w_I_specify=off  y_w_I_priority=None  y_w_I=0  y_w_I_nominal_specify=off  y_w_I_nominal_unit=1  y_w_I_nominal_value=1  HR_I_specify=off  HR_I_priority=None  HR_I=0  HR_I_nominal_specify=off  HR_I_nominal_unit=1  HR_I_nominal_value=1  x_g_I_specify=off  x_g_I_priority=High  x_g_I=0  x_g_I_nominal_specify=off  x_g_I_nominal_unit=1  x_g_I_nominal_value=1  y_g_I_specify=off  y_g_I_priority=None  y_g_I=0  y_g_I_nominal_specify=off  y_g_I_nominal_unit=1  y_g_I_nominal_value=1
      settings: SourceProductBaseCode=SS
  wall_hx : fl_lib/Moist Air/Elements/Pipe (MA)  length=12 m  area=2.5*2.5 m^2  Dh=2.5 m  length_add=0.1 m  roughness=15e-6 m  Re_lam=2000  Re_tur=4000  shape_factor=64  Nu_lam=3.66  RH_ws=1  time_constant=1e-3 s  moisture_trace_gas_source=foundation.enum.moisture_trace_gas_source.none  moisture_source_spec=foundation.enum.moisture_source_spec.vapor  moisture_mass_flow=0 kg/s  moisture_temperature_spec=foundation.enum.temperature_spec.atmospheric  moisture_temperature=293.15 K  trace_gas_mass_flow=0 kg/s  trace_gas_temperature_spec=foundation.enum.temperature_spec.atmospheric  trace_gas_temperature=293.15 K  p_I_specify=off  p_I_priority=High  p_I=0.101325 MPa  p_I_nominal_specify=off  p_I_nominal_unit=MPa  p_I_nominal_value=1  T_I_specify=off  T_I_priority=Low  T_I=box_start_temp degC  T_I_nominal_specify=off  T_I_nominal_unit=K  T_I_nominal_value=1  RH_I_specify=on  RH_I_priority=Low  RH_I=0.5  RH_I_nominal_specify=off  RH_I_nominal_unit=1  RH_I_nominal_value=1  x_w_I_specify=off  x_w_I_priority=None  x_w_I=0  x_w_I_nominal_specify=off  x_w_I_nominal_unit=1  x_w_I_nominal_value=1  y_w_I_specify=off  y_w_I_priority=None  y_w_I=0  y_w_I_nominal_specify=off  y_w_I_nominal_unit=1  y_w_I_nominal_value=1  HR_I_specify=off  HR_I_priority=None  HR_I=0  HR_I_nominal_specify=off  HR_I_nominal_unit=1  HR_I_nominal_value=1  x_g_I_specify=off  x_g_I_priority=High  x_g_I=0  x_g_I_nominal_specify=off  x_g_I_nominal_unit=1  x_g_I_nominal_value=1  y_g_I_specify=off  y_g_I_priority=None  y_g_I=0  y_g_I_nominal_specify=off  y_g_I_nominal_unit=1  y_g_I_nominal_value=1
      settings: SourceProductBaseCode=SS
  Air_out : PMIOPort  Side=Left
  Air_in : PMIOPort  Port=2  Side=Left
  Ambient : PMIOPort  Port=3  Side=Right
  Tcargo_meas : Outport
  wires:
  Constant4/1 -> Simulink-PS Converter4/1
  Constant3/1 -> Simulink-PS Converter5/1
  Constant2/1 -> Simulink-PS Converter6/1
  PS-Simulink Converter/1 -> Tcargo_meas/1
  Transfer Fcn (with initial outputs)/1 -> Gain3/1
  Gain3/1 -> Simulink-PS Converter2/1
  heat_pct/1 -> Transfer Fcn (with initial outputs)/1
  connections:
  Simulink-PS Converter6/RConn1 -- ambient_air/RConn4
  Simulink-PS Converter4/RConn1 -- ambient_air/RConn2
  cargo_2_air_ht/RConn1 -- Tcargo Sensor/LConn1 -- Cargo/LConn1
  Cargo_hx/LConn2 -- cargo_2_air_ht/LConn1
  Flow Resistance (MA)/RConn1 -- ambient_air/LConn1
  Simulink-PS Converter5/RConn1 -- ambient_air/RConn3
  Cargo_hx/RConn1 -- Natural convection mass flow/RConn1 -- cargo_flow_resitance/RConn1 -- Moist Air Properties (MA)/RConn1
  cargo_flow_resitance/LConn1 -- Flow Resistance (MA)/LConn1 -- heating_hx/LConn1
  Tcargo Sensor/RConn1 -- Thermal Reference1/LConn1
  PS-Simulink Converter/LConn1 -- Tcargo Sensor/RConn2
  Cargo_hx/LConn1 -- wall_hx/RConn1
  Air_out/RConn1 -- Natural convection mass flow/LConn1 -- wall_hx/LConn1
  ambient_2_air_ht/LConn1 -- wall_hx/LConn2
  ambient_2_air_ht/RConn1 -- Controlled Heat Flow Rate Source/RConn2 -- ambient_temp/LConn1 -- Ambient/RConn1
  ambient_temp/RConn1 -- Thermal Reference2/LConn1
  ambient_temp/RConn2 -- ambient_air/RConn1
  Air_in/RConn1 -- heating_hx/RConn1
  Simulink-PS Converter2/RConn1 -- Controlled Heat Flow Rate Source/RConn1
  heating_hx/LConn2 -- Controlled Heat Flow Rate Source/LConn1

== system eTRU_prototype_2/Cond_throttle ==
  Vcond : Inport
  Gain4 : Gain  Gain=(((0.005/2)^2)*pi)/100*2
  RefSensor : Subsystem
      settings: PortSchema="{\"entries\":[{\"content\":{\"sides\":[{\"content\":{\"connectorIds\":[\"LConn1\",\"Out1\"]},\"type\":\"ConnectorPlacement.EquallySpacedRectSide\",\"uuid\":\"384ca129-c08e-4242-8b56-38a57a5275bd\"},{\"content\":{\"connectorIds\":[\"RConn1\"],\"side\":\"RIGHT\"},\"type\":\"ConnectorPlacement.EquallySpacedRectSide\",\"uuid\":\"d8d27130-51db-4533-93b1-df7418a29f3a\"},{\"content\":{\"connectorIds\":[],\"side\":\"TOP\"},\"type\":\"ConnectorPlacement.EquallySpacedRectSide\",\"uuid\":\"67192aad-d15e-443e-8c24-a3a889184c8d\"},{\"content\":{\"connectorIds\":[],\"side\":\"BOTTOM\"},\"type\":\"ConnectorPlacement.EquallySpacedRectSide\",\"uuid\":\"18e5bc3a-5c8d-47f7-9803-91861ffb04f2\"}]},\"type\":\"ConnectorPlacement.EquallySpacedConnector\",\"uuid\":\"971e7a76-7cfc-4fb4-bbb6-a40c097b0bda\"}],\"packageUris\":[\"http://schema.mathworks.com/mf0/Connector/19700101\"],\"version\":\"1.0\"}"
  Simulink-PS Converter4 : nesl_utility/Simulink-PS Converter  PhysicalDomain=network_engine_domain  SubClassName=ps_input  LeftPortType=input  RightPortType=output  PseudoPeriodic=off  Frequencies=[]  NoiseDistribution=none  NoiseParameters=[]  Unit=m^2  AffineConversion=off  FilteringAndDerivatives=zero  SimscapeFilterOrder=1  InputFilterTimeConstant=0.001  UdotUserProvided=1
      settings: SourceProductBaseCode=PW,SS
  Transfer Fcn (with initial outputs)2 : simulink_extras/Additional Linear/Transfer Fcn (with initial outputs)  N=[1]  D="[1  1]"  Y0=0  U0=0
  Valve : fl_lib/Two-Phase Fluid/Elements/Variable Local Restriction (2P)  min_area=10e-10 mm^2  max_area=100 mm^2  area=(20/2)^2*pi mm^2  Cd=0.64  B_lam=0.999
      settings: SourceProductBaseCode=SS  InternalSimscapePortConfiguration="{\"Bottom\":[],\"Left\":[{\"id\":\"A\",\"label\":\"A\",\"type\":\"foundation.two_phase_fluid.two_phase_fluid\"},{\"id\":\"area_in\",\"label\":\"AR\",\"type\":\"input\"}],\"Right\":[{\"id\":\"B\",\"label\":\"B\",\"type\":\"foundation.two_phase_fluid.two_phase_fluid\"}],\"Top\":[]}"
  In : PMIOPort  Side=Left
  Out : PMIOPort  Port=2  Side=Right
  RefOutMeas : Outport
  wires:
  Transfer Fcn (with initial outputs)2/1 -> Gain4/1
  Gain4/1 -> Simulink-PS Converter4/1
  Vcond/1 -> Transfer Fcn (with initial outputs)2/1
  RefSensor/1(meas_out) -> RefOutMeas/1
  connections:
  Simulink-PS Converter4/RConn1 -- Valve/LConn2
  In/RConn1 -- Valve/LConn1
  Valve/RConn1 -- RefSensor/LConn1
  RefSensor/RConn1 -- Out/RConn1

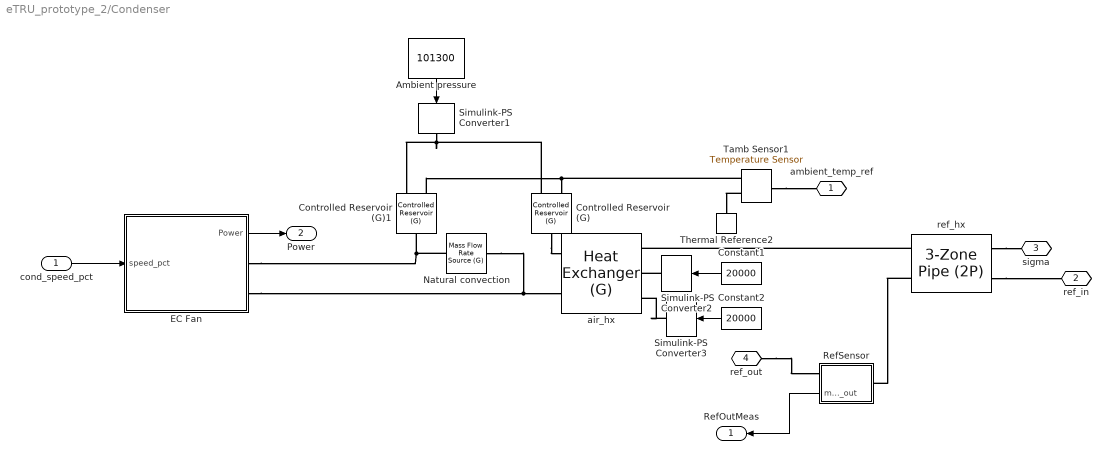
== system eTRU_prototype_2/Condenser ==
  cond_speed_pct : Inport
  Ambient pressure : Constant  Value=101300
  Constant1 : Constant  Value=20000
  Constant2 : Constant  Value=20000
  Controlled Reservoir (G) : fl_lib/Gas/Elements/Controlled Reservoir (G)  area_A=1 m^2
      settings: SourceProductBaseCode=SS  InternalSimscapePortConfiguration="{\"Bottom\":[],\"Left\":[{\"id\":\"A\",\"label\":\"A\",\"type\":\"foundation.gas.gas\"}],\"Right\":[{\"id\":\"T_in\",\"label\":\"T\",\"type\":\"input\"},{\"id\":\"p_in\",\"label\":\"P\",\"type\":\"input\"}],\"Top\":[]}"
  Controlled Reservoir (G)1 : fl_lib/Gas/Elements/Controlled Reservoir (G)  area_A=0.25 m^2
      settings: SourceProductBaseCode=SS  InternalSimscapePortConfiguration="{\"Bottom\":[],\"Left\":[{\"id\":\"A\",\"label\":\"A\",\"type\":\"foundation.gas.gas\"}],\"Right\":[{\"id\":\"T_in\",\"label\":\"T\",\"type\":\"input\"},{\"id\":\"p_in\",\"label\":\"P\",\"type\":\"input\"}],\"Top\":[]}"
  EC Fan : Subsystem
      mask help:
      | Model of EC Fan with air flow and power consumption based on 2D table look-up.
      | Speed and pressure difference is used as table look-up input
      | The data is stored in the file EC_FanData.m that is loaded via model callback.
      | Full speed 100% is 3060 rpm
      |
      | Input:
      | Fan Speed [%] Speed reference
      | Pdiff [Pa]  pressure difference
      |
      | Output:
      | Power [Watt]Power consumption
      | Air_in, Air_out Simscape port for volumetric airflow rate
  Natural convection : fl_lib/Gas/Sources/Mass Flow Rate Source (G)  power_spec=foundation.enum.power_spec.none  mass_flow=0.1 kg/s  area_A=1 m^2  area_B=1 m^2
      settings: SourceProductBaseCode=SS  InternalSimscapePortConfiguration="{\"Bottom\":[],\"Left\":[{\"id\":\"A\",\"label\":\"A\",\"type\":\"foundation.gas.gas\"}],\"Right\":[{\"id\":\"B\",\"label\":\"B\",\"type\":\"foundation.gas.gas\"}],\"Top\":[]}"
  RefSensor : Subsystem
  Simulink-PS Converter1 : nesl_utility/Simulink-PS Converter  PhysicalDomain=network_engine_domain  SubClassName=ps_input  LeftPortType=input  RightPortType=output  PseudoPeriodic=off  Frequencies=[]  NoiseDistribution=none  NoiseParameters=[]  Unit=Pa  AffineConversion=off  FilteringAndDerivatives=zero  SimscapeFilterOrder=1  InputFilterTimeConstant=0.001  UdotUserProvided=1
      settings: SourceProductBaseCode=PW,SS
  Simulink-PS Converter2 : nesl_utility/Simulink-PS Converter  PhysicalDomain=network_engine_domain  SubClassName=ps_input  LeftPortType=input  RightPortType=output  PseudoPeriodic=off  Frequencies=[]  NoiseDistribution=none  NoiseParameters=[]  Unit=W/K  AffineConversion=off  FilteringAndDerivatives=zero  SimscapeFilterOrder=1  InputFilterTimeConstant=0.001  UdotUserProvided=1
      settings: SourceProductBaseCode=PW,SS
  Simulink-PS Converter3 : nesl_utility/Simulink-PS Converter  PhysicalDomain=network_engine_domain  SubClassName=ps_input  LeftPortType=input  RightPortType=output  PseudoPeriodic=off  Frequencies=[]  NoiseDistribution=none  NoiseParameters=[]  Unit=W/(m^2 *K)  AffineConversion=off  FilteringAndDerivatives=zero  SimscapeFilterOrder=1  InputFilterTimeConstant=0.001  UdotUserProvided=1
      settings: SourceProductBaseCode=PW,SS
  Tamb Sensor1 : fl_lib/Thermal/Thermal Sensors/Temperature Sensor
  Thermal Reference2 : fl_lib/Thermal/Thermal Elements/Thermal Reference
  air_hx : SimscapeFluids_lib/Fluid Network Interfaces/Heat Exchangers/Heat Exchanger (G)  hex_type=fluids.interfaces.enum.flow_arrangement_spec.cross_flow  shell_num=1  cross_type=fluids.interfaces.enum.cross_flow_heat_exchanger_G_spec.unmixed_unmixed  NTU_TLU=[.5, 1, 2, 3, 4, 5]  CR_TLU=[0, .25, .5, .75, 1]  eff_TLU=[.3, .3, .3, .3, .3; .6, .55, .5, .47, .43; .85, .76, .68, .61, .55; .94, .83, .72, .65, .58; .98, .86, .75, .66, .58; .99, .86, .75, .66, .58]  R_wall=1.6e-4 K/W  min_flow_area_1=0.1 m^2  Dh_press_1=1 m  gas_volume_1=0.5 m^3  Re_lam_1=2000  Re_tur_1=4000  pressure_loss_spec_1=fluids.interfaces.enum.pressure_loss_spec.constant  pressure_loss_coeff_1=0.1  length_press_1=1 m  length_add_1=0.1 m  roughness_1=15e-6 m  Re_friction_TLU_1=[400, 1000, 1500, 3000, 4000, 6000, 10000, 20000, 40000, 60000, 100000, 100000000]  friction_factor_TLU_1=[.264, .112, .071, .0417, .0387, .0268, .025, .0232, .0226, .022, .0214, .0214]  shape_factor_1=64  Re_Euler_TLU_1=[50, 500, 1000, 2000]  Euler_TLU_1=[4.4505, .6864, .4791, .3755]  heat_transfer_spec_1=fluids.interfaces.enum.heat_transfer_spec.constant  heat_transfer_area_1=3 m^2  heat_coeff_1=10000 W/(m^2 * K)  length_heat_1=1 m  Nu_lam_1=3.66  Re_Colburn_TLU_1=[100, 150, 1000]  Colburn_factor_TLU_1=[.019, .013, .002]  Re_Nu_TLU_1=[100, 150, 1000]  Pr_Nu_TLU_1=[1, 10]  Nu_TLU_1=[3.72, 4.21; 3.75, 4.44; 4.21, 7.15]  fouling_factor_1=1e-4 m^2*K/W  mdot_threshold_1=1e-6 kg/s  min_heat_coeff_1=5 W/(m^2 * K)  heat_transfer_area_2=10 m^2  fouling_factor_2=1e-4 m^2*K/W  min_heat_coeff_2=40 W/(m^2 * K)  T0_1=293.15 K  p0_1=0.101325 MPa  mdot1_TLU=[.3, .5, .6, .7, 1, 1.4, 1.9, 2.3] kg/s  mdot2_TLU=[.3, .5, 1, 1.3, 1.7, 2, 2.6, 3.3] kg/s  SD_TLU=[.324, .3533, .404, .4253, .4333, .4373, .4453, .4533; .3813, .424, .496, .5307, .544, .5547, .5693, .5787; .4267, .4827, .5813, .6173, .6413, .6573, .672, .6827; .4613, .528, .64, .6987, .7267, .7467, .7707, .7853; .5533, .6467, .8227, .928, .9853, 1.0187, 1.0653, 1.0973; .58, .688, .8853, 1.0147, 1.08, 1.124, 1.176, 1.2147; .624, .7467, .992, 1.148, 1.244, 1.304, 1.3773, 1.4267; .656, .7907, 1.0667, 1.26, 1.376, 1.452, 1.548, 1.612] kW/K  Q_check=fluids.interfaces.enum.SD_max_check.warning  mdot_dp_TLU_1=[.3, .5, 1, 1.5, 2, 2.5] kg/s  p_diff_TLU_1=[3, 5, 10, 25, 35, 50] * 1e-3 MPa  T_ref_in_1=293.15 K  p_ref_in_1=0.101325 MPa  area_1=0.01 m^2
      settings: SourceProductBaseCode=SH  InternalSimscapePortConfiguration="{\"Bottom\":[],\"Left\":[{\"id\":\"A1\",\"label\":\"A1\",\"type\":\"foundation.gas.gas\"},{\"id\":\"B1\",\"label\":\"B1\",\"type\":\"foundation.gas.gas\"}],\"Right\":[{\"id\":\"H2\",\"label\":\"H2\",\"type\":\"foundation.thermal.thermal\"},{\"id\":\"C2\",\"label\":\"C2\",\"type\":\"input\"},{\"id\":\"HC2\",\"label\":\"HC2\",\"type\":\"input\"}],\"Top\":[]}"
  ref_hx : SimscapeFluids_lib/Two-Phase Fluid/Pipes & Fittings/3-Zone Pipe (2P)  length=4*1.6 m  area=(0.006/2)^2*pi*15 m^2  Dh=0.006 m  length_add=0.5 m  roughness=0.1 mm  Re_lam=2000  Re_tur=4000  shape_factor=64  hc_ext=4000 W/(m^2*K)  wall_thickness=1.5 mm  k_wall=390 W/(m*K)  c_wall=390 J/(K*kg)  rho_wall=9e3 kg/m^3  fin_ratio_ext=20  eta_fin_ext=0.5  fin_ratio_int=0.1  eta_fin_int=0.5  Nu_lam=3.66  energy_spec=foundation.enum.energy_spec.quality  p_init=start_pressure_high bar  T_init=ambient_temp degC  x_init=0.2  alpha_init=0.5  h_init=1500 kJ/kg  u_init=1500 kJ/kg
      settings: SourceProductBaseCode=SH  InternalSimscapePortConfiguration="{\"Bottom\":[],\"Left\":[{\"id\":\"A\",\"label\":\"A\",\"type\":\"foundation.two_phase_fluid.two_phase_fluid\"},{\"id\":\"H\",\"label\":\"H\",\"type\":\"foundation.thermal.thermal\"}],\"Right\":[{\"id\":\"B\",\"label\":\"B\",\"type\":\"foundation.two_phase_fluid.two_phase_fluid\"},{\"id\":\"Z\",\"label\":\"Z\",\"type\":\"output\"}],\"Top\":[]}"
  ambient_temp_ref : PMIOPort  Side=Left
  ref_in : PMIOPort  Port=2  Side=Left
  sigma : PMIOPort  Port=3  Side=Right
  ref_out : PMIOPort  Port=4  Side=Right
  RefOutMeas : Outport
  Power : Outport  Port=2
  wires:
  Ambient pressure/1 -> Simulink-PS Converter1/1
  Constant1/1 -> Simulink-PS Converter2/1
  cond_speed_pct/1 -> EC Fan/1(speed_pct)
  Constant2/1 -> Simulink-PS Converter3/1
  EC Fan/1(Power) -> Power/1
  RefSensor/1(meas_out) -> RefOutMeas/1
  connections:
  Tamb Sensor1/RConn2 -- Controlled Reservoir (G)1/RConn1 -- Controlled Reservoir (G)/RConn1
  Controlled Reservoir (G)/LConn1 -- air_hx/LConn1
  ref_hx/LConn2 -- air_hx/RConn1
  Simulink-PS Converter2/RConn1 -- air_hx/RConn2
  Simulink-PS Converter1/RConn1 -- Controlled Reservoir (G)1/RConn2 -- Controlled Reservoir (G)/RConn2
  Simulink-PS Converter3/RConn1 -- air_hx/RConn3
  Tamb Sensor1/RConn1 -- Thermal Reference2/LConn1
  ref_hx/RConn1 -- ref_in/RConn1
  ref_hx/RConn2 -- sigma/RConn1
  Tamb Sensor1/LConn1 -- ambient_temp_ref/RConn1
  ref_hx/LConn1 -- RefSensor/LConn1
  ref_out/RConn1 -- RefSensor/RConn1
  EC Fan/RConn2 -- Natural convection/LConn1 -- air_hx/LConn2
  EC Fan/RConn1 -- Natural convection/RConn1 -- Controlled Reservoir (G)1/LConn1
